simulink model "model2"  (R2021b)
settings: Solver=VariableStepAuto  StartTime=0.0  StopTime=10.0  RelTol=1e-3
settings Model: Creator=Clement_Wu  LastModifiedBy=Clement_Wu

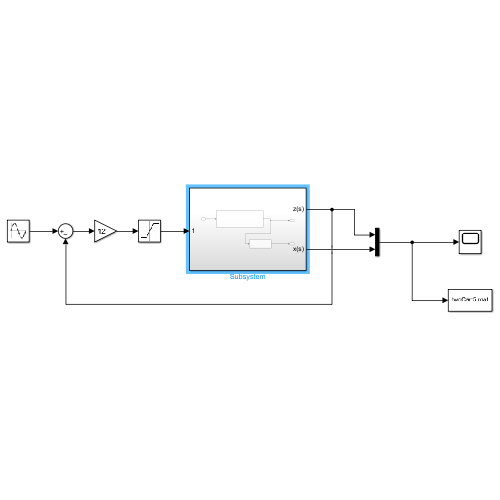
[thumbnail: Simulink's stored preview of the top-level diagram]
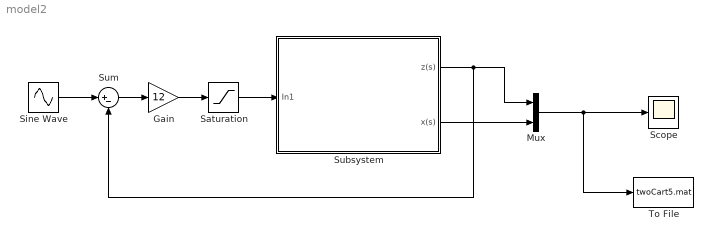
== system model2 ==
  Gain : Gain  Gain=12
  Mux : Mux  Inputs=2
  Saturation : Saturate  UpperLimit=2.5  LowerLimit=-2.5
  Scope : Scope
  Sine Wave : Sin  Amplitude=0.4  Frequency=16.5250  SampleTime=0
  Subsystem : Subsystem
  Sum : Sum  Inputs=|+-
  To File : ToFile  Filename=twoCart5.mat  MatrixName=ans5  SaveFormat=Timeseries
  wires:
  Subsystem/1(z(s)) -> Sum/2, Mux/1
  Sum/1 -> Gain/1
  Gain/1 -> Saturation/1
  Sine Wave/1 -> Sum/1
  Saturation/1 -> Subsystem/1(In1)
  Mux/1 -> To File/1, Scope/1
  Subsystem/2(x(s)) -> Mux/2

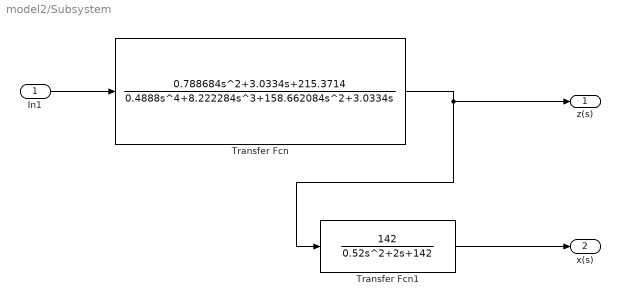
== system model2/Subsystem ==
  In1 : Inport
  Transfer Fcn : TransferFcn  Numerator=[0.788684 3.0334 215.3714]  Denominator=[0.4888 8.222284 158.662084 3.0334 0]
  Transfer Fcn1 : TransferFcn  Numerator=[142]  Denominator=[0.52 2 142]
  z(s) : Outport
  x(s) : Outport  Port=2
  wires:
  Transfer Fcn/1 -> Transfer Fcn1/1, z(s)/1
  Transfer Fcn1/1 -> x(s)/1
  In1/1 -> Transfer Fcn/1
